simulink model "linearController"  (R2024a)
settings: Solver=FixedStepAuto  StartTime=0.0  StopTime=50  FixedStep=.01  RelTol=1e-3
values from neighbouring files (symbols this model uses):
  D2R = pi/180    (= 0.0174532925199)    [IPdynamicsHomoclinicOrbitStabilization.m]    (also in invertedPendulumDynamics.m)
  dtheta0 = 0    [IPdynamicsHomoclinicOrbitStabilization.m]
  dx0 = 0    [IPdynamicsHomoclinicOrbitStabilization.m]
  g = 9.804    [IPdynamicsHomoclinicOrbitStabilization.m]    (also in invertedPendulumDynamics.m = 9.81)
  K = lqr(A,B,Q,R)    [IPdynamicsHomoclinicOrbitStabilization.m]    (also in invertedPendulumDynamics.m = [-31.6228, -22.4894, 87.1251, 18.1589])
  l = 0.2425    [IPdynamicsHomoclinicOrbitStabilization.m]    (also in invertedPendulumDynamics.m = 0.3)
  m = .3    (= 0.3)    [IPdynamicsHomoclinicOrbitStabilization.m]    (also in invertedPendulumDynamics.m)
  M = 1.035052    [IPdynamicsHomoclinicOrbitStabilization.m]    (also in invertedPendulumDynamics.m = 1)
  ml = m*l    (= 0.07275)    [IPdynamicsHomoclinicOrbitStabilization.m]    (also in invertedPendulumDynamics.m = 0.09)
  ml2 = ml*l    (= 0.017641875)    [IPdynamicsHomoclinicOrbitStabilization.m]    (also in invertedPendulumDynamics.m = 0.027)
  R2D = 180/pi    (= 57.2957795131)    [IPdynamicsHomoclinicOrbitStabilization.m]    (also in invertedPendulumDynamics.m)
  x0 = 0    [IPdynamicsHomoclinicOrbitStabilization.m]
libraries: vrlib x3
settings Model: PauseTimes=0.386  SnapshotBufferSize=6  SnapshotInterval=5  Creator=rahelmizrahi  LastModifiedBy=rahelmizrahi

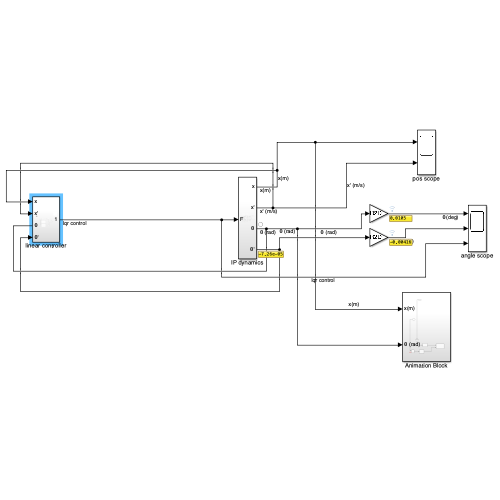
[thumbnail: Simulink's stored preview of the top-level diagram]
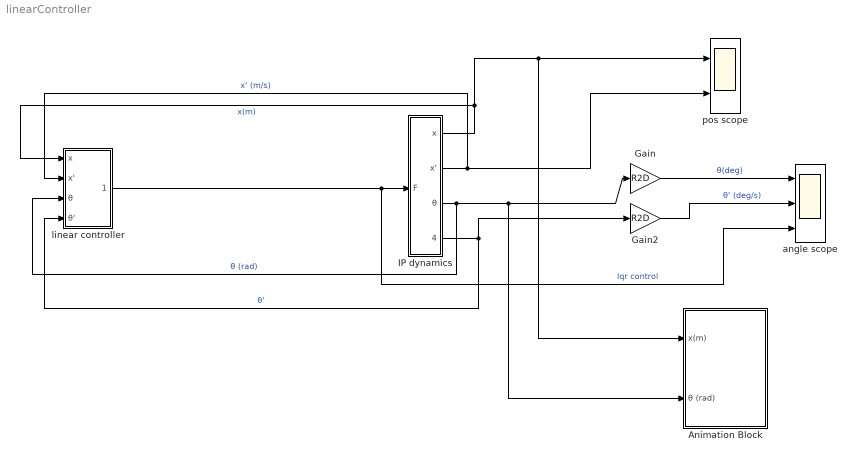
== system linearController ==
  Animation Block : Subsystem
  Gain : Gain  Gain=R2D
  Gain2 : Gain  Gain=R2D
  IP dynamics : Subsystem
  angle scope : Scope  NumInputPorts=3
  linear controller : Subsystem
  pos scope : Scope  NumInputPorts=2
  wires:
  linear controller/1(Output1) -> angle scope/3, IP dynamics/1(F)  "lqr control"
  IP dynamics/4(θ') -> linear controller/4(θ'), Gain2/1  "θ'"
  Gain/1 -> angle scope/1  "θ(deg)"
  IP dynamics/2(x') -> pos scope/2, linear controller/2(x')  "x' (m/s)"
  Gain2/1 -> angle scope/2  "θ' (deg/s)"
  IP dynamics/3(θ) -> linear controller/3(θ), Animation Block/2(θ (rad)), Gain/1  "θ (rad)"
  IP dynamics/1(x) -> Animation Block/1(x(m)), pos scope/1, linear controller/1(x)  "x(m)"

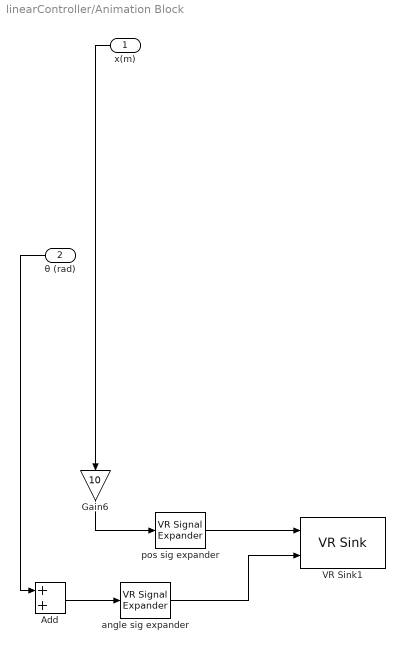
== system linearController/Animation Block ==
  x(m) : Inport
  θ (rad) : Inport  Port=2
  Add : Sum
  Gain6 : Gain  Gain=10
  VR Sink1 : vrlib/VR Sink  InstantiateOnLoad=on  SampleTime=0.1  ViewEnable=on  RemoteChange=off  RemoteView=off  FieldsWritten=cart.translation.3.1.1.double#joint.rotation.4.1.1.double  WorldFileName=/Users/rahelmizrahi/Downloads/upload 2/Inverted_pendulum12.wrl  AutoView=on  VideoDimensions=[]  AllowVariableSize=off
  angle sig expander : vrlib/VR Signal Expander  outwidth=4  outidx=4
  pos sig expander : vrlib/VR Signal Expander  outwidth=3  outidx=1
  wires:
  θ (rad)/1 -> Add/1
  pos sig expander/1 -> VR Sink1/1
  Add/1 -> angle sig expander/1
  ? -> Add/2
  Gain6/1 -> pos sig expander/1
  angle sig expander/1 -> VR Sink1/2
  x(m)/1 -> Gain6/1

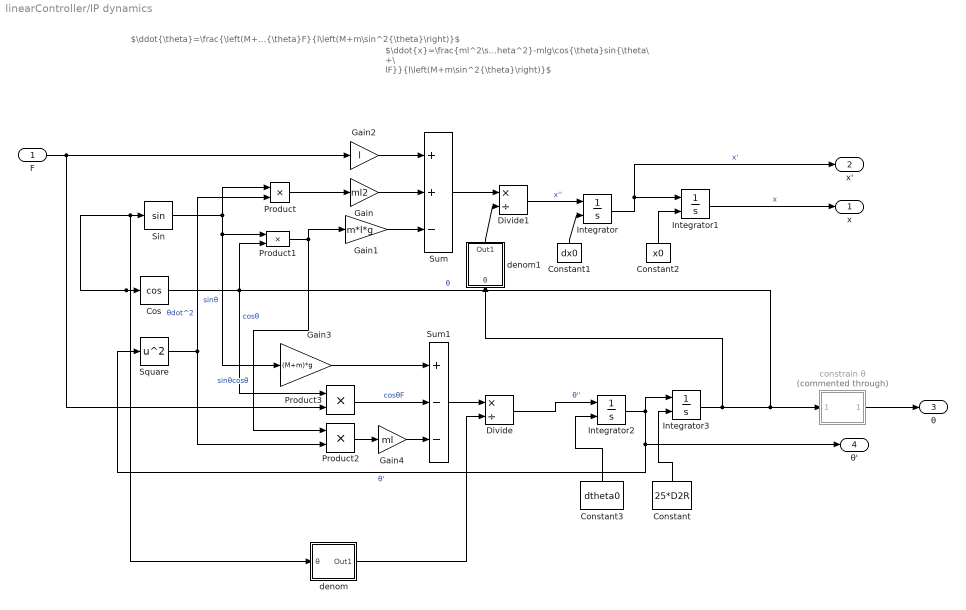
== system linearController/IP dynamics ==
  note: $\ddot{\theta}=\frac{\left(M+m\right)g\sin{\theta-ml\sin{\theta}\cos{\theta}\dot{\theta^2}}-\cos{\theta}F}{l\left(M+m\sin^2{\theta}\right)}$
  note: $\ddot{x}=\frac{ml^2\sin{\theta}\dot{\theta^2}-mlg\cos{\theta}sin{\theta\ +\ lF}}{l\left(M+m\sin^2{\theta}\right)}$
  F : Inport
  Constant : Constant  Value=25*D2R
  Constant1 : Constant  Value=dx0
  Constant2 : Constant  Value=x0
  Constant3 : Constant  Value=dtheta0
  Cos : Trigonometry  Operator=cos
  Divide : Product  Inputs=*/
  Divide1 : Product  Inputs=*/
  Gain : Gain  Gain=ml2
  Gain1 : Gain  Gain=m*l*g
  Gain2 : Gain  Gain=l
  Gain3 : Gain  Gain=(M+m)*g
  Gain4 : Gain  Gain=ml
  Integrator : Integrator  InitialConditionSource=external
  Integrator1 : Integrator  InitialConditionSource=external
  Integrator2 : Integrator  InitialConditionSource=external
  Integrator3 : Integrator  InitialConditionSource=external  WrappedStateUpperValue=2*pi  WrappedStateLowerValue=0
  Product{,1..3} (4 alike) : Product
  Sin : Trigonometry
  Square : Math  Operator=square
  Sum : Sum  Inputs=++-
  Sum1 : Sum  Inputs=+--
  constrain θ : MATLAB Function  Commented=through  TreatAsAtomicUnit=on
  denom : Subsystem
  denom1 : Subsystem
  x : Outport
  x' : Outport  Port=2
  θ : Outport  Port=3
  θ' : Outport  Port=4
  wires:
  Product/1 -> Gain/1
  Sum1/1 -> Divide/1
  F/1 -> Product3/2, Gain2/1
  Gain2/1 -> Sum/1
  Product1/1 -> Product2/1, Gain1/1  "sinθcosθ"
  Product3/1 -> Sum1/2  "cosθF"
  Gain1/1 -> Sum/3
  Integrator1/1 -> x/1  "x"
  Square/1 -> Product/2, Product2/2  "θdot^2"
  Cos/1 -> Product1/2, Product3/1  "cosθ"
  Integrator2/1 -> Integrator3/1, θ'/1, Square/1  "θ'"
  Integrator3/1 -> denom1/1(θ), denom/1(θ), Sin/1, Cos/1, constrain θ/1("theta ")  "θ"
  Gain3/1 -> Sum1/1
  Gain/1 -> Sum/2
  Product2/1 -> Gain4/1
  Sin/1 -> Gain3/1, Product1/1, Product/1  "sinθ"
  Integrator/1 -> x'/1, Integrator1/1  "x'"
  Sum/1 -> Divide1/1
  Gain4/1 -> Sum1/3
  Constant/1 -> Integrator3/2
  Constant1/1 -> Integrator/2
  Constant2/1 -> Integrator1/2
  Constant3/1 -> Integrator2/2
  Divide/1 -> Integrator2/1  "θ''"
  denom/1(Out1) -> Divide/2
  Divide1/1 -> Integrator/1  "x''"
  denom1/1(Out1) -> Divide1/2
  constrain θ/1(theta) -> θ/1

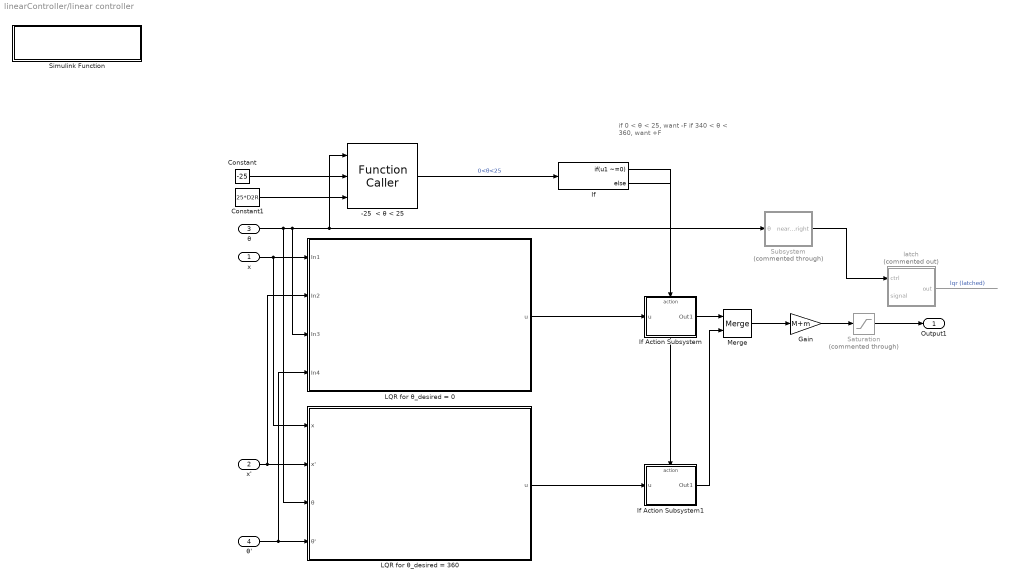
== system linearController/linear controller ==
  note: if 0 < θ < 25, want -F
      | if 340 < θ < 360, want +F
  x : Inport
  x' : Inport  Port=2
  θ : Inport  Port=3
  θ' : Inport  Port=4
  -25  < θ < 25 : FunctionCaller  FunctionPrototype=out = between(input,min,max)  InputArgumentSpecifications=double(1), double(1), double(1)  OutputArgumentSpecifications=boolean(1)
  Constant : Constant  Value=-25
  Constant1 : Constant  Value=25*D2R
  Gain : Gain  Gain=M+m
  If : If  IfExpression=u1 ~=0
  If Action Subsystem : Subsystem  TreatAsAtomicUnit=on
  If Action Subsystem1 : Subsystem  TreatAsAtomicUnit=on
  LQR for θ_desired = 0 : Subsystem
  LQR for θ_desired = 360 : Subsystem
  Merge : Merge
  Saturation : Saturate  Commented=through  UpperLimit=5  LowerLimit=-5
  Simulink Function : Subsystem  TreatAsAtomicUnit=on
  Subsystem : Subsystem  Commented=through
  latch : Subsystem  Commented=on
  Output1 : Outport
  wires:
  Merge/1 -> Gain/1
  If Action Subsystem/1(Out1) -> Merge/1
  x/1 -> LQR for θ_desired = 0/1(In1), LQR for θ_desired = 360/1(x)
  x'/1 -> LQR for θ_desired = 0/2(In2), LQR for θ_desired = 360/2(x')
  LQR for θ_desired = 360/1(u) -> If Action Subsystem1/1(u)
  -25  < θ < 25/1 -> If/1  "0<θ<25"
  θ'/1 -> LQR for θ_desired = 0/4(In4), LQR for θ_desired = 360/4(θ')
  If/1 -> If Action Subsystem/Action
  If/2 -> If Action Subsystem1/Action
  θ/1 -> Subsystem/1(θ), -25  < θ < 25/1, LQR for θ_desired = 0/3(In3), LQR for θ_desired = 360/3(θ)
  If Action Subsystem1/1(Out1) -> Merge/2
  Constant1/1 -> -25  < θ < 25/3
  Constant/1 -> -25  < θ < 25/2
  Subsystem/1(near_upright) -> latch/1(ctrl)
  latch/1(out) -> ?  "lqr (latched)"
  Saturation/1 -> Output1/1
  Gain/1 -> Saturation/1
  LQR for θ_desired = 0/1(u) -> If Action Subsystem/1(u)

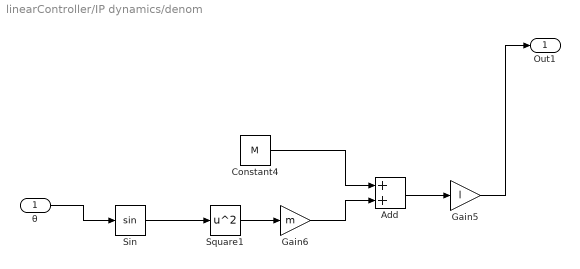
== system linearController/IP dynamics/denom ==
  θ : Inport
  Add : Sum
  Constant4 : Constant  Value=M
  Gain5 : Gain  Gain=l
  Gain6 : Gain  Gain=m
  Sin : Trigonometry
  Square1 : Math  Operator=square
  Out1 : Outport
  wires:
  Gain5/1 -> Out1/1
  Square1/1 -> Gain6/1
  θ/1 -> Sin/1
  Constant4/1 -> Add/1
  Add/1 -> Gain5/1
  Gain6/1 -> Add/2
  Sin/1 -> Square1/1

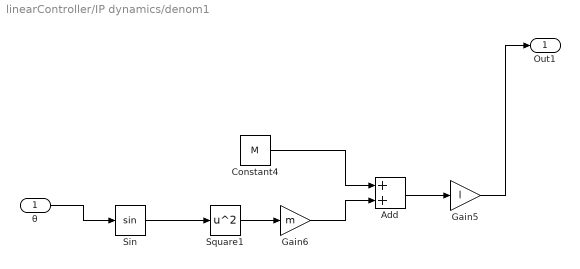
== system linearController/IP dynamics/denom1 ==
  θ : Inport
  Add : Sum
  Constant4 : Constant  Value=M
  Gain5 : Gain  Gain=l
  Gain6 : Gain  Gain=m
  Sin : Trigonometry
  Square1 : Math  Operator=square
  Out1 : Outport
  wires:
  Gain5/1 -> Out1/1
  Square1/1 -> Gain6/1
  θ/1 -> Sin/1
  Constant4/1 -> Add/1
  Add/1 -> Gain5/1
  Gain6/1 -> Add/2
  Sin/1 -> Square1/1

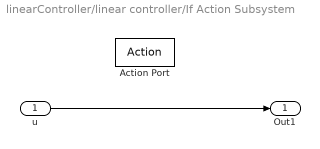
== system linearController/linear controller/If Action Subsystem ==
  u : Inport
  Action Port : ActionPort  ActionPortLabel=if(u1 ~=0)
  Out1 : Outport
  wires:
  u/1 -> Out1/1

== system linearController/linear controller/If Action Subsystem1 ==
  u : Inport
  Action Port : ActionPort  ActionPortLabel=else
  Out1 : Outport
  wires:
  u/1 -> Out1/1

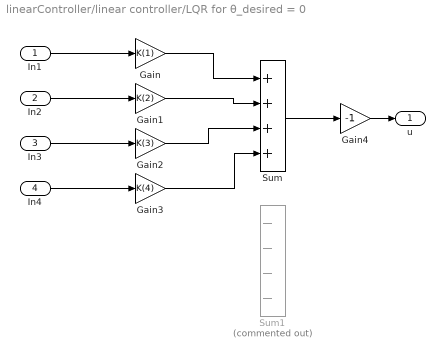
== system linearController/linear controller/LQR for θ_desired = 0 ==
  In1 : Inport
  In2 : Inport  Port=2
  In3 : Inport  Port=3
  In4 : Inport  Port=4
  Gain : Gain  Gain=K(1)
  Gain1 : Gain  Gain=K(2)
  Gain2 : Gain  Gain=K(3)
  Gain3 : Gain  Gain=K(4)
  Gain4 : Gain  Gain=-1
  Sum : Sum  Inputs=++++
  Sum1 : Sum  Commented=on  Inputs=----
  u : Outport
  wires:
  In4/1 -> Gain3/1
  In2/1 -> Gain1/1
  Gain1/1 -> Sum/2
  Gain3/1 -> Sum/4
  Sum/1 -> Gain4/1
  Gain2/1 -> Sum/3
  In3/1 -> Gain2/1
  In1/1 -> Gain/1
  Gain/1 -> Sum/1
  Gain4/1 -> u/1

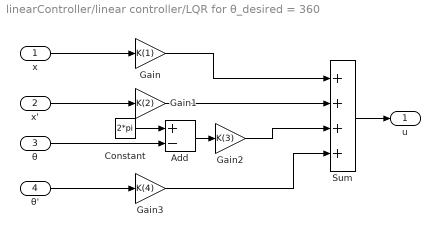
== system linearController/linear controller/LQR for θ_desired = 360 ==
  x : Inport
  x' : Inport  Port=2
  θ : Inport  Port=3
  θ' : Inport  Port=4
  Add : Sum  Inputs=+-
  Constant : Constant  Value=2*pi
  Gain : Gain  Gain=K(1)
  Gain1 : Gain  Gain=K(2)
  Gain2 : Gain  Gain=K(3)
  Gain3 : Gain  Gain=K(4)
  Sum : Sum  Inputs=++++
  u : Outport
  wires:
  θ'/1 -> Gain3/1
  x'/1 -> Gain1/1
  Gain1/1 -> Sum/2
  Gain3/1 -> Sum/4
  Sum/1 -> u/1
  θ/1 -> Add/2
  x/1 -> Gain/1
  Gain/1 -> Sum/1
  Constant/1 -> Add/1
  Add/1 -> Gain2/1
  Gain2/1 -> Sum/3

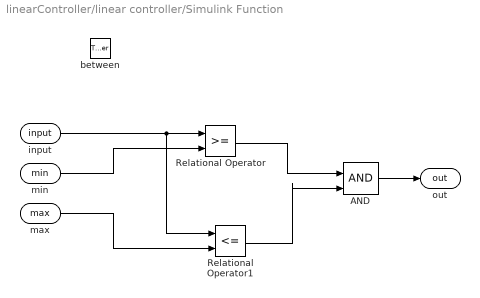
== system linearController/linear controller/Simulink Function ==
  between : TriggerPort  TriggerType=function-call  IsSimulinkFunction=on  FunctionName=between  FunctionVisibility=scoped  VariantControl=(inherit)
  AND : Logic  IconShape=distinctive  AllPortsSameDT=off  OutDataTypeStr=boolean
  Relational Operator : RelationalOperator  OutDataTypeStr=boolean  RndMeth=Simplest  InputSameDT=off
  Relational Operator1 : RelationalOperator  Operator=<=  OutDataTypeStr=boolean  RndMeth=Simplest  InputSameDT=off
  input : ArgIn  DisableCoverage=on  ArgumentName=input
  min : ArgIn  Port=2  ArgumentName=min
  max : ArgIn  Port=3  ArgumentName=max
  out : ArgOut  DisableCoverage=on  OutDataTypeStr=boolean  ArgumentName=out
  wires:
  input/1 -> Relational Operator1/1, Relational Operator/1
  Relational Operator/1 -> AND/1
  Relational Operator1/1 -> AND/2
  AND/1 -> out/1
  min/1 -> Relational Operator/2
  max/1 -> Relational Operator1/2

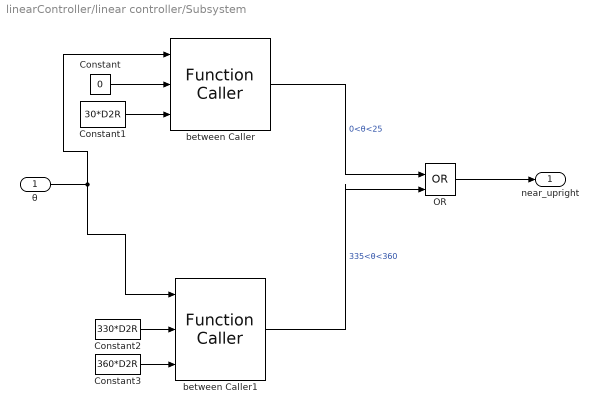
== system linearController/linear controller/Subsystem ==
  θ : Inport
  Constant : Constant  Value=0
  Constant1 : Constant  Value=30*D2R
  Constant2 : Constant  Value=330*D2R
  Constant3 : Constant  Value=360*D2R
  OR : Logic  Operator=OR  IconShape=distinctive  AllPortsSameDT=off  OutDataTypeStr=boolean
  between Caller : FunctionCaller  FunctionPrototype=out = between(input,min,max)  InputArgumentSpecifications=double(1), double(1), double(1)  OutputArgumentSpecifications=boolean(1)
  between Caller1 : FunctionCaller  FunctionPrototype=out = between(input,min,max)  InputArgumentSpecifications=double(1), double(1), double(1)  OutputArgumentSpecifications=boolean(1)
  near_upright : Outport
  wires:
  θ/1 -> between Caller1/1, between Caller/1
  between Caller1/1 -> OR/2  "335<θ<360"
  Constant3/1 -> between Caller1/3
  Constant1/1 -> between Caller/3
  between Caller/1 -> OR/1  "0<θ<25"
  Constant/1 -> between Caller/2
  Constant2/1 -> between Caller1/2
  OR/1 -> near_upright/1

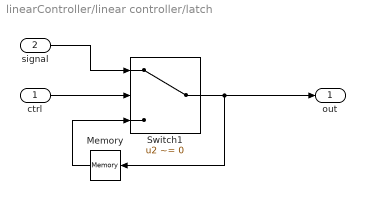
== system linearController/linear controller/latch ==
  ctrl : Inport
  signal : Inport  Port=2
  Memory : Memory
  Switch1 : Switch  Criteria=u2 ~= 0  SaturateOnIntegerOverflow=off  InputSameDT=off
  out : Outport
  wires:
  signal/1 -> Switch1/1
  Memory/1 -> Switch1/3
  Switch1/1 -> out/1, Memory/1
  ctrl/1 -> Switch1/2

== matlab function linearController/IP dynamics/constrain θ ==
  data: theta input; theta output
function theta = constrain(theta)
D2R = pi/180;
    if (theta > 0) && (theta < 360*D2R)
        theta = theta; 
    elseif theta > 360*D2R
        while theta > 360*D2R
            theta = theta - 360*D2R;
        end
    elseif theta < 0
        while theta < 0
            theta = theta + 360*D2R;
        end
    end
end
